simulink model "CoETS_StTrqLimCalc"  (R2016b)
settings: configuration reference "CodeGenConfigSet" (kept outside this file)
values from neighbouring files (symbols this model uses):
  CoETS_nTrqRatMin_C = Calibration.Parameter    [init_CoETS_StTrqLimCalc.m]    (also in init_CoETS_StTrqLimCalc_SIL.m = Simulink.Parameter)
  CoETS_trqDiffMaxLim_C = Calibration.Parameter    [init_CoETS_StTrqLimCalc.m]    (also in init_CoETS_StTrqLimCalc_SIL.m = Simulink.Parameter)
  CoETS_trqInrCurrMinLim_C = Calibration.Parameter    [init_CoETS_StTrqLimCalc.m]    (also in init_CoETS_StTrqLimCalc_SIL.m = Simulink.Parameter)
  PRC_100 = fi(100,Prc_100_rate)    [init_CoETS_StTrqLimCalc.m]    (also in init_CoETS_StTrqLimCalc_SIL.m)
  PRC_ZERO = fi(0,Prc_100_rate)    [init_CoETS_StTrqLimCalc.m]    (also in init_CoETS_StTrqLimCalc_SIL.m)
  Rail_stLimDetSetPoint_C = Calibration.Parameter    [init_CoETS_StTrqLimCalc.m]    (also in init_CoETS_StTrqLimCalc_SIL.m = Simulink.Parameter)
libraries: simulink x68, CXLib x2
settings Model: Creator=Wollf  LastModifiedBy=Wollf
settings ConfigSetRef: SourceLocation=Base Workspace

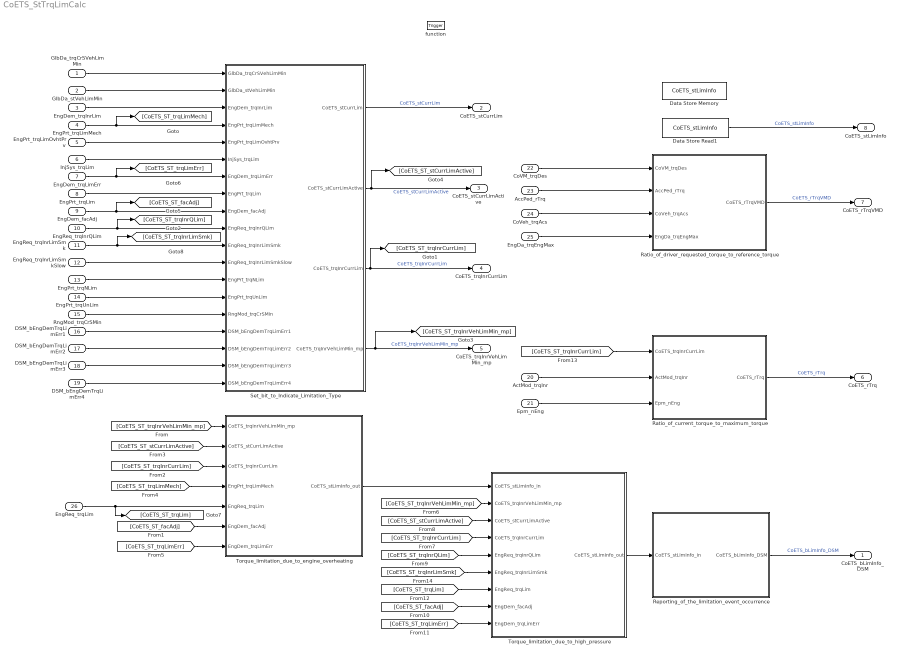
== system CoETS_StTrqLimCalc ==
  GlbDa_trqCrSVehLimMin : Inport  Tag=Nm  Description=current limitation torque from GlbDa on torque level crankshaft  OutMin=-3276.8  OutMax=3276.7  OutDataTypeStr=Trq_Nm
  GlbDa_stVehLimMin : Inport  Description=Current limitation state from GlbDa  Port=2  OutMin=0  OutMax=255  OutDataTypeStr=State_uint8
  EngDem_trqInrLim : Inport  Tag=Nm  Description=Resulting limiting torque (inner engine torque)  Port=3  OutMin=-3276.8  OutMax=3276.7  OutDataTypeStr=Trq_Nm
  EngPrt_trqLimMech : Inport  Tag=Nm  Description=Resulting limiting torque for engine mechanics protection (inner engine torque)  Port=4  OutMin=-3276.8  OutMax=3276.7  OutDataTypeStr=Trq_Nm
  EngPrt_trqLimOvhtPrv : Inport  Tag=Nm  Description=Torque limitation value for engine protection from overheating  Port=5  OutMin=-3276.8  OutMax=3276.7  OutDataTypeStr=Trq_Nm
  InjSys_trqLim : Inport  Tag=Nm  Description=Torque limitation of injection system  Port=6  OutMin=-3276.8  OutMax=3276.7  OutDataTypeStr=Trq_Nm
  EngDem_trqLimErr : Inport  Tag=Nm  Description=Substitute limiting torque in the event of an error  Port=7  OutMin=-3276.8  OutMax=3276.7  OutDataTypeStr=Trq_Nm
  EngPrt_trqLim : Inport  Tag=Nm  Description=Limitation torque for engine mechanic protection by torque limitation (as inner engine torque)  Port=8  OutMin=-3276.8  OutMax=3276.7  OutDataTypeStr=Trq_Nm
  EngDem_facAdj : Inport  Description=EEPROM adjustment value for correction of the limiting torque  Port=9  OutMin=-10  OutMax=10  OutDataTypeStr=Factor
  EngReq_trqInrQLim : Inport  Tag=Nm  Description=Limiting torque due to limitation quantities (except smoke limitation)  Port=10  OutMin=-3276.8  OutMax=3276.7  OutDataTypeStr=Trq_Nm
  EngReq_trqInrLimSmk : Inport  Tag=Nm  Description=Limiting torque smoke limit  Port=11  OutMin=-3276.8  OutMax=3276.7  OutDataTypeStr=Trq_Nm
  EngReq_trqInrLimSmkSlow : Inport  Tag=Nm  Description=Limiting torque smoke limit of slow path  Port=12  OutMin=-3276.8  OutMax=3276.7  OutDataTypeStr=Trq_Nm
  EngPrt_trqNLim : Inport  Tag=Nm  Description=Limiting torque for protection from excessive engine speed  Port=13  OutMin=-3276.8  OutMax=3276.7  OutDataTypeStr=Trq_Nm
  EngPrt_trqUnLim : Inport  Tag=Nm  Description=Enabled torque from the maximum power manager  Port=14  OutMin=-3276.8  OutMax=3276.7  OutDataTypeStr=Trq_Nm
  RngMod_trqCrSMin : Inport  Tag=Nm  Description=minimal crankshaft torque  Port=15  OutMin=-3276.8  OutMax=3276.7  OutDataTypeStr=Trq_Nm
  DSM_bEngDemTrqLimErr1 : Inport  Description=FId for Engine demand Torque Limitation due to System error  Port=16  OutMin=0  OutMax=1  OutDataTypeStr=boolean
  DSM_bEngDemTrqLimErr2 : Inport  Description=FId for Engine demand Torque Limitation due to System error  Port=17  OutMin=0  OutMax=1  OutDataTypeStr=boolean
  DSM_bEngDemTrqLimErr3 : Inport  Description=FId for Engine demand Torque Limitation due to System error  Port=18  OutMin=0  OutMax=1  OutDataTypeStr=boolean
  DSM_bEngDemTrqLimErr4 : Inport  Description=FId for Engine demand Torque Limitation due to System error  Port=19  OutMin=0  OutMax=1  OutDataTypeStr=boolean
  ActMod_trqInr : Inport  Tag=Nm  Description=Current, back-calculated inner engine torque  Port=20  OutMin=-3276.8  OutMax=3276.7  OutDataTypeStr=Trq_Nm
  Epm_nEng : Inport  Tag=rpm  Description=Engine speed  Port=21  OutMin=0  OutMax=6000  OutDataTypeStr=EngSpeed_rpm
  CoVM_trqDes : Inport  Tag=Nm  Description=Propulsion torque order after ESP-torque intervention coordination (wheel torque)  Port=22  OutMin=-3000  OutMax=3000  OutDataTypeStr=Trq_Nm
  AccPed_rTrq : Inport  Description=Total drive train ratio of engine - wheel  Port=23  OutMin=-327  OutMax=327  OutDataTypeStr=TransRatio
  CoVeh_trqAcs : Inport  Tag=Nm  Description=message for demand of accessories  Port=24  OutMin=-3276.8  OutMax=3276.7  OutDataTypeStr=Trq_Nm
  EngDa_trqEngMax : Inport  Tag=Nm  Description=Maximum engine output torque  Port=25  OutMin=-3276.8  OutMax=3276.7  OutDataTypeStr=Trq_Nm
  EngReq_trqLim : Inport  Tag=Nm  Description=Resulting limiting torque from engine specifications  Port=26  OutMin=-3276.8  OutMax=3276.7  OutDataTypeStr=Trq_Nm
  function : TriggerPort  TriggerType=function-call  VariantControl=Variant
  Data Store Memory : DataStoreMemory  DataStoreName=CoETS_stLimInfo  ReadBeforeWriteMsg=warning  WriteAfterWriteMsg=warning  WriteAfterReadMsg=warning  ShowAdditionalParam=off
  Data Store Read1 : DataStoreRead  DataStoreName=CoETS_stLimInfo
  Ratio_of_current_torque_to_maximum_torque : Subsystem
  Ratio_of_driver_requested_torque_to_reference_torque : Subsystem
  Reporting_of_the_limitation_event_occurrence : Subsystem
  Set_bit_to_Indicate_Limitation_Type : Subsystem
  Torque_limitation_due_to_engine_overheating : Subsystem
  Torque_limitation_due_to_high_pressure : Subsystem
  CoETS_bLimInfo_DSM : Outport  Description=DFC of CoETS_bLimInfo  OutMin=0  OutMax=1  OutDataTypeStr=boolean
  CoETS_stCurrLim : Outport  Description=status word for type of lowest limitations  Port=2  OutMin=0  OutMax=65535  OutDataTypeStr=State_uint16
  CoETS_stCurrLimActive : Outport  Description=status of active minimum of limitation torques  Port=3  OutMin=0  OutMax=65535  OutDataTypeStr=State_uint16
  CoETS_trqInrCurrLim : Outport  Tag=Nm  Description=Current lowest limitation torque (inner engine torque)  Port=4  OutMin=-3276.8  OutMax=3276.7  OutDataTypeStr=Trq_Nm
  CoETS_trqInrVehLimMin_mp : Outport  Tag=Nm  Description="Coordinated limitation torque of vehicle functions  (inner torque)"  Port=5  OutMin=-3276.8  OutMax=3276.7  OutDataTypeStr=Trq_Nm
  CoETS_rTrq : Outport  Tag=%  Description=Calculated load value  Port=6  OutMin=-300  OutMax=300  OutDataTypeStr=Prc_100_rate
  CoETS_rTrqVMD : Outport  Tag=%  Description=Ratio of driver requested torque to engine reference torque  Port=7  OutMin=-300  OutMax=300  OutDataTypeStr=Prc_100_rate
  CoETS_stLimInfo : Outport  Description=Status information on working torque limitation  Port=8  OutMin=0  OutMax=255  OutDataTypeStr=State_uint8
  wires:
  RngMod_trqCrSMin/1 -> Set_bit_to_Indicate_Limitation_Type/15(RngMod_trqCrSMin)
  AccPed_rTrq/1 -> Ratio_of_driver_requested_torque_to_reference_torque/2(AccPed_rTrq)
  Ratio_of_driver_requested_torque_to_reference_torque/1("CoETS_rTrqVMD ") -> CoETS_rTrqVMD/1  "CoETS_rTrqVMD"
  CoVM_trqDes/1 -> Ratio_of_driver_requested_torque_to_reference_torque/1(CoVM_trqDes)
  EngDa_trqEngMax/1 -> Ratio_of_driver_requested_torque_to_reference_torque/4(EngDa_trqEngMax)
  CoVeh_trqAcs/1 -> Ratio_of_driver_requested_torque_to_reference_torque/3(CoVeh_trqAcs)
  Ratio_of_current_torque_to_maximum_torque/1(CoETS_rTrq) -> CoETS_rTrq/1  "CoETS_rTrq"
  EngReq_trqInrLimSmk/1 -> Set_bit_to_Indicate_Limitation_Type/11(EngReq_trqInrLimSmk), [CoETS_ST_trqInrLimSmk]
  EngPrt_trqLim/1 -> Set_bit_to_Indicate_Limitation_Type/8(EngPrt_trqLim)
  InjSys_trqLim/1 -> Set_bit_to_Indicate_Limitation_Type/6("InjSys_trqLim ")
  EngDem_facAdj/1 -> Set_bit_to_Indicate_Limitation_Type/9(EngDem_facAdj), [CoETS_ST_facAdj]
  EngDem_trqLimErr/1 -> Set_bit_to_Indicate_Limitation_Type/7(EngDem_trqLimErr), [CoETS_ST_trqLimErr]
  EngPrt_trqUnLim/1 -> Set_bit_to_Indicate_Limitation_Type/14(EngPrt_trqUnLim)
  EngPrt_trqNLim/1 -> Set_bit_to_Indicate_Limitation_Type/13(EngPrt_trqNLim)
  Set_bit_to_Indicate_Limitation_Type/2(CoETS_stCurrLimActive) -> CoETS_stCurrLimActive/1, [CoETS_ST_stCurrLimActive]  "CoETS_stCurrLimActive"
  EngReq_trqInrLimSmkSlow/1 -> Set_bit_to_Indicate_Limitation_Type/12(EngReq_trqInrLimSmkSlow)
  GlbDa_stVehLimMin/1 -> Set_bit_to_Indicate_Limitation_Type/2(GlbDa_stVehLimMin)
  EngReq_trqInrQLim/1 -> Set_bit_to_Indicate_Limitation_Type/10(EngReq_trqInrQLim), [CoETS_ST_trqInrQLim]
  EngDem_trqInrLim/1 -> Set_bit_to_Indicate_Limitation_Type/3(EngDem_trqInrLim)
  GlbDa_trqCrSVehLimMin/1 -> Set_bit_to_Indicate_Limitation_Type/1(GlbDa_trqCrSVehLimMin)
  EngPrt_trqLimOvhtPrv/1 -> Set_bit_to_Indicate_Limitation_Type/5("EngPrt_trqLimOvhtPrv ")
  Set_bit_to_Indicate_Limitation_Type/1(CoETS_stCurrLim) -> CoETS_stCurrLim/1  "CoETS_stCurrLim"
  EngPrt_trqLimMech/1 -> Set_bit_to_Indicate_Limitation_Type/4(EngPrt_trqLimMech), [CoETS_ST_trqLimMech]
  [CoETS_ST_trqInrCurrLim] -> Ratio_of_current_torque_to_maximum_torque/1(CoETS_trqInrCurrLim)
  Set_bit_to_Indicate_Limitation_Type/3(CoETS_trqInrCurrLim) -> CoETS_trqInrCurrLim/1, [CoETS_ST_trqInrCurrLim]  "CoETS_trqInrCurrLim"
  [CoETS_ST_trqInrCurrLim] -> Torque_limitation_due_to_engine_overheating/3(CoETS_trqInrCurrLim)
  Set_bit_to_Indicate_Limitation_Type/4(CoETS_trqInrVehLimMin_mp) -> CoETS_trqInrVehLimMin_mp/1, [CoETS_ST_trqInrVehLimMin_mp]  "CoETS_trqInrVehLimMin_mp"
  [CoETS_ST_trqInrVehLimMin_mp] -> Torque_limitation_due_to_engine_overheating/1(CoETS_trqInrVehLimMin_mp)
  [CoETS_ST_stCurrLimActive] -> Torque_limitation_due_to_engine_overheating/2(CoETS_stCurrLimActive)
  [CoETS_ST_trqLimMech] -> Torque_limitation_due_to_engine_overheating/4(EngPrt_trqLimMech)
  EngReq_trqLim/1 -> Torque_limitation_due_to_engine_overheating/5(EngReq_trqLim), [CoETS_ST_trqLim]
  [CoETS_ST_facAdj] -> Torque_limitation_due_to_engine_overheating/6(EngDem_facAdj)
  [CoETS_ST_trqLimErr] -> Torque_limitation_due_to_engine_overheating/7(EngDem_trqLimErr)
  [CoETS_ST_trqInrVehLimMin_mp] -> Torque_limitation_due_to_high_pressure/2(CoETS_trqInrVehLimMin_mp)
  [CoETS_ST_stCurrLimActive] -> Torque_limitation_due_to_high_pressure/3(CoETS_stCurrLimActive)
  [CoETS_ST_trqInrCurrLim] -> Torque_limitation_due_to_high_pressure/4(CoETS_trqInrCurrLim)
  [CoETS_ST_trqInrQLim] -> Torque_limitation_due_to_high_pressure/5(EngReq_trqInrQLim)
  [CoETS_ST_facAdj] -> Torque_limitation_due_to_high_pressure/8(EngDem_facAdj)
  [CoETS_ST_trqLimErr] -> Torque_limitation_due_to_high_pressure/9(EngDem_trqLimErr)
  [CoETS_ST_trqLim] -> Torque_limitation_due_to_high_pressure/7(EngReq_trqLim)
  [CoETS_ST_trqInrLimSmk] -> Torque_limitation_due_to_high_pressure/6(EngReq_trqInrLimSmk)
  Torque_limitation_due_to_engine_overheating/1("CoETS_stLimInfo_out ") -> Torque_limitation_due_to_high_pressure/1(CoETS_stLimInfo_in)
  Torque_limitation_due_to_high_pressure/1("CoETS_stLimInfo_out ") -> Reporting_of_the_limitation_event_occurrence/1(CoETS_stLimInfo_in)
  Reporting_of_the_limitation_event_occurrence/1(CoETS_bLimInfo_DSM) -> CoETS_bLimInfo_DSM/1  "CoETS_bLimInfo_DSM"
  DSM_bEngDemTrqLimErr1/1 -> Set_bit_to_Indicate_Limitation_Type/16(DSM_bEngDemTrqLimErr1)
  DSM_bEngDemTrqLimErr2/1 -> Set_bit_to_Indicate_Limitation_Type/17(DSM_bEngDemTrqLimErr2)
  DSM_bEngDemTrqLimErr3/1 -> Set_bit_to_Indicate_Limitation_Type/18(DSM_bEngDemTrqLimErr3)
  DSM_bEngDemTrqLimErr4/1 -> Set_bit_to_Indicate_Limitation_Type/19(DSM_bEngDemTrqLimErr4)
  ActMod_trqInr/1 -> Ratio_of_current_torque_to_maximum_torque/2(ActMod_trqInr)
  Epm_nEng/1 -> Ratio_of_current_torque_to_maximum_torque/3(Epm_nEng)
  Data Store Read1/1 -> CoETS_stLimInfo/1  "CoETS_stLimInfo"

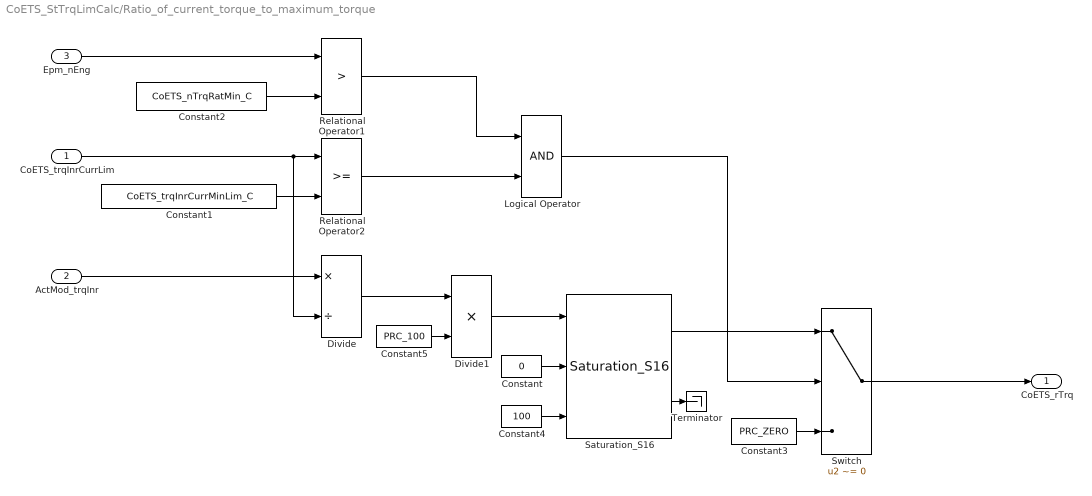
== system CoETS_StTrqLimCalc/Ratio_of_current_torque_to_maximum_torque ==
  CoETS_trqInrCurrLim : Inport
  ActMod_trqInr : Inport  Port=2
  Epm_nEng : Inport  Port=3
  Constant : Constant  Value=0  OutDataTypeStr=Inherit: Inherit via back propagation
  Constant1 : Constant  Value=CoETS_trqInrCurrMinLim_C
  Constant2 : Constant  Value=CoETS_nTrqRatMin_C
  Constant3 : Constant  Value=PRC_ZERO  OutDataTypeStr=Inherit: Inherit via back propagation
  Constant4 : Constant  Value=100  OutDataTypeStr=Inherit: Inherit via back propagation
  Constant5 : Constant  Value=PRC_100  OutDataTypeStr=uint8
  Divide : Product  Inputs=*/  OutDataTypeStr=Accpedal_rate  SaturateOnIntegerOverflow=on
  Divide1 : Product  Inputs=**  OutDataTypeStr=Inherit: Inherit via back propagation  SaturateOnIntegerOverflow=on
  Logical Operator : Logic  OutDataTypeStr=boolean
  Relational Operator1 : RelationalOperator  Operator=>  OutDataTypeStr=boolean  RndMeth=Nearest  InputSameDT=on
  Relational Operator2 : RelationalOperator  OutDataTypeStr=boolean  RndMeth=Nearest  InputSameDT=on
  Saturation_S16 : CXLib/Saturation_S16
  Switch : Switch  Criteria=u2 ~= 0  SaturateOnIntegerOverflow=on  InputSameDT=on
  Terminator : Terminator
  CoETS_rTrq : Outport
  wires:
  CoETS_trqInrCurrLim/1 -> Relational Operator2/1, Divide/2
  Constant2/1 -> Relational Operator1/2
  Epm_nEng/1 -> Relational Operator1/1
  Constant1/1 -> Relational Operator2/2
  Relational Operator1/1 -> Logical Operator/1
  Relational Operator2/1 -> Logical Operator/2
  Logical Operator/1 -> Switch/2
  Constant3/1 -> Switch/3
  ActMod_trqInr/1 -> Divide/1
  Divide/1 -> Divide1/1
  Constant/1 -> Saturation_S16/2
  Constant4/1 -> Saturation_S16/3
  Saturation_S16/2 -> Terminator/1
  Saturation_S16/1 -> Switch/1
  Switch/1 -> CoETS_rTrq/1
  Constant5/1 -> Divide1/2
  Divide1/1 -> Saturation_S16/1

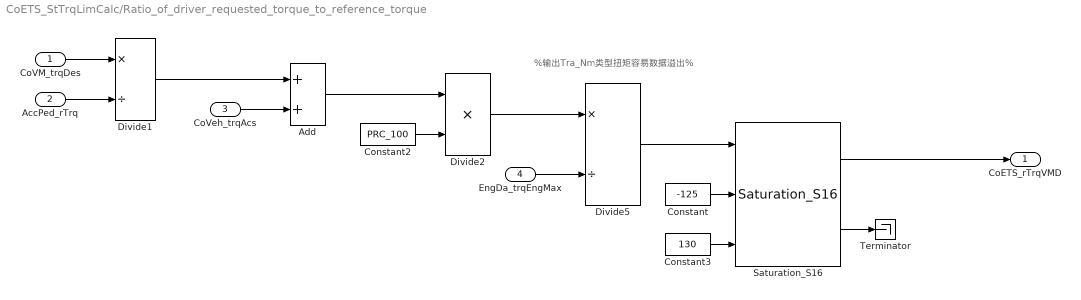
== system CoETS_StTrqLimCalc/Ratio_of_driver_requested_torque_to_reference_torque ==
  note: %输出Tra_Nm类型扭矩容易数据溢出%
  CoVM_trqDes : Inport
  AccPed_rTrq : Inport  Port=2
  CoVeh_trqAcs : Inport  Port=3
  EngDa_trqEngMax : Inport  Port=4
  Add : Sum  SaturateOnIntegerOverflow=on  InputSameDT=on
  Constant : Constant  Value=-125  OutDataTypeStr=Inherit: Inherit via back propagation
  Constant2 : Constant  Value=PRC_100  OutDataTypeStr=uint8
  Constant3 : Constant  Value=130  OutDataTypeStr=Inherit: Inherit via back propagation
  Divide1 : Product  Inputs=*/  OutDataTypeStr=Trq_Nm  SaturateOnIntegerOverflow=on
  Divide2 : Product  Inputs=**  OutDataTypeStr=int32  SaturateOnIntegerOverflow=on
  Divide5 : Product  Inputs=*/  OutDataTypeStr=Inherit: Inherit via back propagation  SaturateOnIntegerOverflow=on
  Saturation_S16 : CXLib/Saturation_S16
  Terminator : Terminator
  "CoETS_rTrqVMD " : Outport
  wires:
  AccPed_rTrq/1 -> Divide1/2
  Divide1/1 -> Add/1
  CoVeh_trqAcs/1 -> Add/2
  Add/1 -> Divide2/1
  Constant2/1 -> Divide2/2
  EngDa_trqEngMax/1 -> Divide5/2
  Divide5/1 -> Saturation_S16/1
  Constant/1 -> Saturation_S16/2
  Constant3/1 -> Saturation_S16/3
  Saturation_S16/1 -> "CoETS_rTrqVMD "/1
  Saturation_S16/2 -> Terminator/1
  CoVM_trqDes/1 -> Divide1/1
  Divide2/1 -> Divide5/1

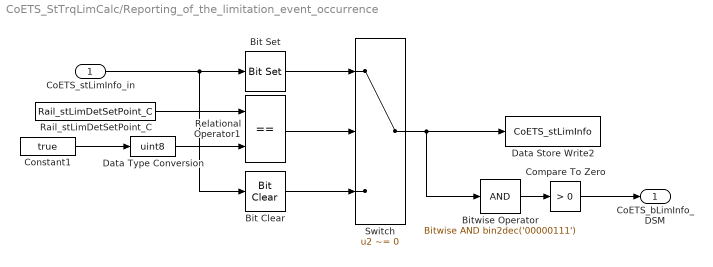
== system CoETS_StTrqLimCalc/Reporting_of_the_limitation_event_occurrence ==
  CoETS_stLimInfo_in : Inport
  Bit Clear : simulink/Logic and Bit Operations/Bit Clear  iBit=2
  Bit Set : simulink/Logic and Bit Operations/Bit Set  iBit=2
  Bitwise Operator : simulink/Logic and Bit Operations/Bitwise Operator  logicop=AND  UseBitMask=on  BitMask=bin2dec('00000111')  BitMaskRealWorld=Stored Integer
  Compare To Zero : simulink/Logic and Bit Operations/Compare To Zero  relop=>  OutDataTypeStr=boolean
  Constant1 : Constant  Value=true  OutDataTypeStr=boolean
  Data Store Write2 : DataStoreWrite  DataStoreName=CoETS_stLimInfo
  Data Type Conversion : DataTypeConversion  OutDataTypeStr=uint8
  Rail_stLimDetSetPoint_C : Constant  Value=Rail_stLimDetSetPoint_C
  Relational Operator1 : RelationalOperator  Operator===  OutDataTypeStr=boolean  RndMeth=Nearest  InputSameDT=on
  Switch : Switch  Criteria=u2 ~= 0  InputSameDT=on
  CoETS_bLimInfo_DSM : Outport
  wires:
  Constant1/1 -> Data Type Conversion/1
  Relational Operator1/1 -> Switch/2
  CoETS_stLimInfo_in/1 -> Bit Clear/1, Bit Set/1
  Bit Set/1 -> Switch/1
  Bit Clear/1 -> Switch/3
  Rail_stLimDetSetPoint_C/1 -> Relational Operator1/1
  Switch/1 -> Data Store Write2/1, Bitwise Operator/1
  Bitwise Operator/1 -> Compare To Zero/1
  Compare To Zero/1 -> CoETS_bLimInfo_DSM/1
  Data Type Conversion/1 -> Relational Operator1/2

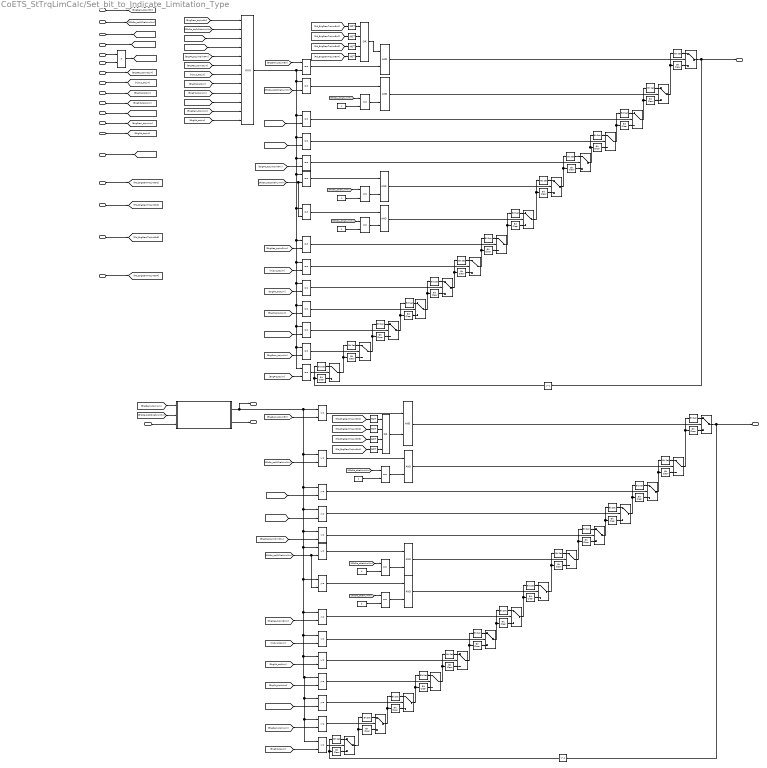
== system CoETS_StTrqLimCalc/Set_bit_to_Indicate_Limitation_Type ==
  note: FId must be a uint16 constant
  GlbDa_trqCrSVehLimMin : Inport
  GlbDa_stVehLimMin : Inport  Port=2
  EngDem_trqInrLim : Inport  Port=3
  EngPrt_trqLimMech : Inport  Port=4
  "EngPrt_trqLimOvhtPrv " : Inport  Port=5
  "InjSys_trqLim " : Inport  Port=6
  EngDem_trqLimErr : Inport  Port=7
  EngPrt_trqLim : Inport  Port=8
  EngDem_facAdj : Inport  Port=9
  EngReq_trqInrQLim : Inport  Port=10
  EngReq_trqInrLimSmk : Inport  Port=11
  EngReq_trqInrLimSmkSlow : Inport  Port=12
  EngPrt_trqNLim : Inport  Port=13
  EngPrt_trqUnLim : Inport  Port=14
  RngMod_trqCrSMin : Inport  Port=15
  DSM_bEngDemTrqLimErr1 : Inport  Port=16
  DSM_bEngDemTrqLimErr2 : Inport  Port=17
  DSM_bEngDemTrqLimErr3 : Inport  Port=18
  DSM_bEngDemTrqLimErr4 : Inport  Port=19
  Bit Clear1 : simulink/Logic and Bit Operations/Bit Clear  iBit=0
  Bit Clear12 : simulink/Logic and Bit Operations/Bit Clear  iBit=10
  Bit Clear14 : simulink/Logic and Bit Operations/Bit Clear  iBit=11
  Bit Clear16 : simulink/Logic and Bit Operations/Bit Clear  iBit=12
  Bit Clear18 : simulink/Logic and Bit Operations/Bit Clear  iBit=13
  Bit Clear2 : simulink/Logic and Bit Operations/Bit Clear  iBit=6
  Bit Clear20 : simulink/Logic and Bit Operations/Bit Clear  iBit=14
  Bit Clear3 : simulink/Logic and Bit Operations/Bit Clear  iBit=1
  Bit Clear4 : simulink/Logic and Bit Operations/Bit Clear  iBit=2
  Bit Clear41 : simulink/Logic and Bit Operations/Bit Clear  iBit=0
  Bit Clear44 : simulink/Logic and Bit Operations/Bit Clear  iBit=10
  Bit Clear46 : simulink/Logic and Bit Operations/Bit Clear  iBit=11
  Bit Clear48 : simulink/Logic and Bit Operations/Bit Clear  iBit=12
  Bit Clear5 : simulink/Logic and Bit Operations/Bit Clear  iBit=3
  Bit Clear50 : simulink/Logic and Bit Operations/Bit Clear  iBit=13
  Bit Clear52 : simulink/Logic and Bit Operations/Bit Clear  iBit=6
  Bit Clear53 : simulink/Logic and Bit Operations/Bit Clear  iBit=14
  Bit Clear54 : simulink/Logic and Bit Operations/Bit Clear  iBit=1
  Bit Clear55 : simulink/Logic and Bit Operations/Bit Clear  iBit=2
  Bit Clear56 : simulink/Logic and Bit Operations/Bit Clear  iBit=3
  Bit Clear57 : simulink/Logic and Bit Operations/Bit Clear  iBit=5
  Bit Clear58 : simulink/Logic and Bit Operations/Bit Clear  iBit=7
  Bit Clear59 : simulink/Logic and Bit Operations/Bit Clear  iBit=8
  Bit Clear6 : simulink/Logic and Bit Operations/Bit Clear  iBit=5
  Bit Clear60 : simulink/Logic and Bit Operations/Bit Clear  iBit=9
  Bit Clear7 : simulink/Logic and Bit Operations/Bit Clear  iBit=7
  Bit Clear8 : simulink/Logic and Bit Operations/Bit Clear  iBit=8
  Bit Clear9 : simulink/Logic and Bit Operations/Bit Clear  iBit=9
  Bit Set1 : simulink/Logic and Bit Operations/Bit Set  iBit=0
  Bit Set10 : simulink/Logic and Bit Operations/Bit Set  iBit=10
  Bit Set11 : simulink/Logic and Bit Operations/Bit Set  iBit=11
  Bit Set12 : simulink/Logic and Bit Operations/Bit Set  iBit=12
  Bit Set13 : simulink/Logic and Bit Operations/Bit Set  iBit=13
  Bit Set14 : simulink/Logic and Bit Operations/Bit Set  iBit=14
  Bit Set15 : simulink/Logic and Bit Operations/Bit Set  iBit=9
  Bit Set16 : simulink/Logic and Bit Operations/Bit Set  iBit=10
  Bit Set17 : simulink/Logic and Bit Operations/Bit Set  iBit=6
  Bit Set18 : simulink/Logic and Bit Operations/Bit Set  iBit=1
  Bit Set19 : simulink/Logic and Bit Operations/Bit Set  iBit=2
  Bit Set2 : simulink/Logic and Bit Operations/Bit Set  iBit=6
  Bit Set20 : simulink/Logic and Bit Operations/Bit Set  iBit=3
  Bit Set21 : simulink/Logic and Bit Operations/Bit Set  iBit=5
  Bit Set22 : simulink/Logic and Bit Operations/Bit Set  iBit=7
  Bit Set23 : simulink/Logic and Bit Operations/Bit Set  iBit=8
  Bit Set24 : simulink/Logic and Bit Operations/Bit Set  iBit=0
  Bit Set25 : simulink/Logic and Bit Operations/Bit Set  iBit=11
  Bit Set26 : simulink/Logic and Bit Operations/Bit Set  iBit=12
  Bit Set27 : simulink/Logic and Bit Operations/Bit Set  iBit=13
  Bit Set28 : simulink/Logic and Bit Operations/Bit Set  iBit=14
  Bit Set3 : simulink/Logic and Bit Operations/Bit Set  iBit=1
  Bit Set4 : simulink/Logic and Bit Operations/Bit Set  iBit=2
  Bit Set5 : simulink/Logic and Bit Operations/Bit Set  iBit=3
  Bit Set6 : simulink/Logic and Bit Operations/Bit Set  iBit=5
  Bit Set7 : simulink/Logic and Bit Operations/Bit Set  iBit=7
  Bit Set8 : simulink/Logic and Bit Operations/Bit Set  iBit=8
  Bit Set9 : simulink/Logic and Bit Operations/Bit Set  iBit=9
  Constant1 : Constant  OutDataTypeStr=uint8
  Constant12 : Constant  OutDataTypeStr=uint8
  Constant13 : Constant  Value=4  OutDataTypeStr=uint8
  Constant14 : Constant  Value=2  OutDataTypeStr=Inherit: Inherit via back propagation
  Constant2 : Constant  Value=4  OutDataTypeStr=uint8
  Constant3 : Constant  Value=2  OutDataTypeStr=uint8
  Delay : Delay  DelayLength=1  InitialCondition=0
  Delay2 : Delay  DelayLength=1  InitialCondition=0
  Determining_the_current_minimum_of_all_torque_limitations : Subsystem
  Divide : Product  Inputs=**  OutDataTypeStr=Inherit: Inherit via back propagation  SaturateOnIntegerOverflow=on
  Logical Operator{,1..2,4,6..8,16} (8 alike) : Logic  OutDataTypeStr=boolean
  Logical Operator{5,9..11,13..14,17,19} (8 alike) : Logic  Operator=NOT  OutDataTypeStr=boolean
  Logical Operator12 : Logic  Operator=OR  Inputs=4  OutDataTypeStr=boolean
  Logical Operator15 : Logic  Operator=OR  Inputs=4  OutDataTypeStr=boolean
  MinMax : MinMax  Inputs=12  SaturateOnIntegerOverflow=on  InputSameDT=on
  Relational Operator{1..5,7,9,11..17} (14 alike) : RelationalOperator  OutDataTypeStr=boolean  RndMeth=Nearest  InputSameDT=on
  Relational Operator{6,8,10,18..34} (20 alike) : RelationalOperator  Operator===  OutDataTypeStr=boolean  RndMeth=Nearest  InputSameDT=on
  Switch{1..14,29..42} (28 alike) : Switch  Criteria=u2 ~= 0  InputSameDT=on
  CoETS_stCurrLim : Outport
  CoETS_stCurrLimActive : Outport  Port=2
  CoETS_trqInrCurrLim : Outport  Port=3
  CoETS_trqInrVehLimMin_mp : Outport  Port=4
  wires:
  EngDem_trqLimErr/1 -> [EngDem_trqLimErr]
  Bit Set1/1 -> Switch1/1
  Bit Clear1/1 -> Switch1/3
  Logical Operator16/1 -> Switch1/2
  Switch1/1 -> Delay/1, CoETS_stCurrLim/1
  Logical Operator/1 -> Switch3/2
  Bit Set3/1 -> Switch3/1
  Bit Clear3/1 -> Switch3/3
  Bit Set4/1 -> Switch4/1
  Bit Clear4/1 -> Switch4/3
  Relational Operator4/1 -> Switch4/2
  Relational Operator1/1 -> Switch5/2
  Bit Set5/1 -> Switch5/1
  Bit Clear5/1 -> Switch5/3
  Bit Set6/1 -> Switch6/1
  Bit Clear6/1 -> Switch6/3
  Relational Operator5/1 -> Switch6/2
  GlbDa_trqCrSVehLimMin/1 -> [GlbDa_trqCrSVehLimMin]
  Relational Operator3/1 -> Logical Operator/1
  Relational Operator6/1 -> Logical Operator/2
  GlbDa_stVehLimMin/1 -> [GlbDa_stVehLimMin]
  Constant1/1 -> Relational Operator6/2
  EngPrt_trqLimMech/1 -> [EngPrt_trqLimMech]
  EngReq_trqInrLimSmk/1 -> [EngReq_trqInrLimSmk]
  Bit Clear2/1 -> Switch2/3
  Logical Operator1/1 -> Switch2/2
  Relational Operator8/1 -> Logical Operator1/2
  Relational Operator7/1 -> Logical Operator1/1
  Constant2/1 -> Relational Operator8/2
  Bit Set2/1 -> Switch2/1
  Bit Clear7/1 -> Switch7/3
  Logical Operator2/1 -> Switch7/2
  Relational Operator10/1 -> Logical Operator2/2
  Relational Operator9/1 -> Logical Operator2/1
  Bit Set7/1 -> Switch7/1
  Constant3/1 -> Relational Operator10/2
  Bit Set8/1 -> Switch8/1
  Bit Clear8/1 -> Switch8/3
  Relational Operator11/1 -> Switch8/2
  Bit Clear9/1 -> Switch9/3
  Relational Operator12/1 -> Switch9/2
  "InjSys_trqLim "/1 -> [InjSys_trqLim]
  Bit Set15/1 -> Switch9/1
  Bit Clear12/1 -> Switch10/3
  Relational Operator13/1 -> Switch10/2
  EngPrt_trqNLim/1 -> [EngPrt_trqNLim]
  Bit Set16/1 -> Switch10/1
  Bit Clear14/1 -> Switch11/3
  Relational Operator14/1 -> Switch11/2
  EngPrt_trqUnLim/1 -> [EngPrt_trqUnLim]
  Bit Set25/1 -> Switch11/1
  Determining_the_current_minimum_of_all_torque_limitations/1(CoETS_trqInrCurrLim) -> Relational Operator7/1, Relational Operator17/1, Relational Operator16/1, Relational Operator15/1, Relational Operator14/1, Relational Operator13/1, Relational Operator12/1, Relational Operator11/1, Relational Operator9/1, Relational Operator5/1, Relational Operator1/1, Relational Operator4/1, Relational Operator3/1, Relational Operator2/1, CoETS_trqInrCurrLim/1
  Bit Clear16/1 -> Switch12/3
  Relational Operator15/1 -> Switch12/2
  EngReq_trqInrLimSmkSlow/1 -> [EngReq_trqInrLimSmkSlow]
  Bit Set26/1 -> Switch12/1
  Bit Clear18/1 -> Switch13/3
  Relational Operator16/1 -> Switch13/2
  Bit Set27/1 -> Switch13/1
  Bit Clear20/1 -> Switch14/3
  Relational Operator17/1 -> Switch14/2
  Bit Set28/1 -> Switch14/1
  EngDem_trqInrLim/1 -> [EngDem_trqInrLim]
  EngPrt_trqLim/1 -> [EngPrt_trqLim]
  EngDem_facAdj/1 -> Divide/2
  "EngPrt_trqLimOvhtPrv "/1 -> Divide/1
  Divide/1 -> [EngPrt_trqLimOvhtPrv]
  Switch14/1 -> Bit Set27/1, Bit Clear18/1
  Switch13/1 -> Bit Set26/1, Bit Clear16/1
  Switch12/1 -> Bit Set25/1, Bit Clear14/1
  Switch11/1 -> Bit Set16/1, Bit Clear12/1
  Switch10/1 -> Bit Set15/1, Bit Clear9/1
  Switch9/1 -> Bit Clear8/1, Bit Set8/1
  Switch8/1 -> Bit Set7/1, Bit Clear7/1
  Switch7/1 -> Bit Clear2/1, Bit Set2/1
  Switch2/1 -> Bit Clear6/1, Bit Set6/1
  Switch6/1 -> Bit Clear5/1, Bit Set5/1
  Switch5/1 -> Bit Clear4/1, Bit Set4/1
  Switch4/1 -> Bit Clear3/1, Bit Set3/1
  Switch3/1 -> Bit Clear1/1, Bit Set1/1
  Delay/1 -> Bit Set28/1, Bit Clear20/1
  Bit Set24/1 -> Switch29/1
  Bit Clear41/1 -> Switch29/3
  Logical Operator4/1 -> Switch29/2
  Switch29/1 -> CoETS_stCurrLimActive/1, Delay2/1
  Logical Operator6/1 -> Switch36/2
  Bit Set18/1 -> Switch36/1
  Bit Clear54/1 -> Switch36/3
  Bit Set19/1 -> Switch37/1
  Bit Clear55/1 -> Switch37/3
  Relational Operator21/1 -> Switch37/2
  Relational Operator22/1 -> Switch38/2
  Bit Set20/1 -> Switch38/1
  Bit Clear56/1 -> Switch38/3
  Bit Set21/1 -> Switch39/1
  Bit Clear57/1 -> Switch39/3
  Relational Operator23/1 -> Switch39/2
  Relational Operator19/1 -> Logical Operator6/1
  Relational Operator20/1 -> Logical Operator6/2
  Bit Clear52/1 -> Switch35/3
  Logical Operator7/1 -> Switch35/2
  Relational Operator25/1 -> Logical Operator7/2
  Relational Operator24/1 -> Logical Operator7/1
  Bit Set17/1 -> Switch35/1
  Bit Clear58/1 -> Switch40/3
  Logical Operator8/1 -> Switch40/2
  Relational Operator27/1 -> Logical Operator8/2
  Relational Operator26/1 -> Logical Operator8/1
  Bit Set22/1 -> Switch40/1
  Bit Set23/1 -> Switch41/1
  Bit Clear59/1 -> Switch41/3
  Relational Operator28/1 -> Switch41/2
  Bit Clear60/1 -> Switch42/3
  Relational Operator29/1 -> Switch42/2
  Bit Set9/1 -> Switch42/1
  Bit Clear44/1 -> Switch30/3
  Relational Operator30/1 -> Switch30/2
  Bit Set10/1 -> Switch30/1
  Bit Clear46/1 -> Switch31/3
  Relational Operator31/1 -> Switch31/2
  Bit Set11/1 -> Switch31/1
  Bit Clear48/1 -> Switch32/3
  Relational Operator32/1 -> Switch32/2
  Bit Set12/1 -> Switch32/1
  Bit Clear50/1 -> Switch33/3
  Relational Operator33/1 -> Switch33/2
  Bit Set13/1 -> Switch33/1
  Bit Clear53/1 -> Switch34/3
  Relational Operator34/1 -> Switch34/2
  Bit Set14/1 -> Switch34/1
  Switch34/1 -> Bit Set13/1, Bit Clear50/1
  Switch33/1 -> Bit Set12/1, Bit Clear48/1
  Switch32/1 -> Bit Set11/1, Bit Clear46/1
  Switch31/1 -> Bit Set10/1, Bit Clear44/1
  Switch30/1 -> Bit Set9/1, Bit Clear60/1
  Switch42/1 -> Bit Clear59/1, Bit Set23/1
  Switch41/1 -> Bit Set22/1, Bit Clear58/1
  Switch40/1 -> Bit Clear52/1, Bit Set17/1
  Switch35/1 -> Bit Set21/1, Bit Clear57/1
  Switch39/1 -> Bit Clear56/1, Bit Set20/1
  Switch38/1 -> Bit Clear55/1, Bit Set19/1
  Switch37/1 -> Bit Clear54/1, Bit Set18/1
  Switch36/1 -> Bit Clear41/1, Bit Set24/1
  Delay2/1 -> Bit Set14/1, Bit Clear53/1
  EngReq_trqInrQLim/1 -> [EngReq_trqInrQLim]
  [EngDem_trqLimErr] -> MinMax/1
  [GlbDa_trqCrSVehLimMin] -> MinMax/2
  [GlbDa_stVehLimMin] -> Relational Operator20/1
  [EngReq_trqInrLimSmk] -> MinMax/4
  [EngPrt_trqLimOvhtPrv] -> MinMax/5
  [EngReq_trqInrQLim] -> MinMax/6
  [InjSys_trqLim] -> MinMax/7
  [EngPrt_trqNLim] -> MinMax/8
  [EngPrt_trqUnLim] -> MinMax/9
  [EngReq_trqInrLimSmkSlow] -> MinMax/10
  [EngDem_trqInrLim] -> MinMax/11
  [EngPrt_trqLim] -> MinMax/12
  Relational Operator18/1 -> Logical Operator4/2
  MinMax/1 -> Relational Operator21/1, Relational Operator26/1, Relational Operator34/1, Relational Operator33/1, Relational Operator32/1, Relational Operator31/1, Relational Operator30/1, Relational Operator29/1, Relational Operator28/1, Relational Operator24/1, Relational Operator23/1, Relational Operator22/1, Relational Operator19/1, Relational Operator18/2
  [EngDem_trqLimErr] -> Relational Operator18/1
  [GlbDa_trqCrSVehLimMin] -> Relational Operator19/2
  Constant12/1 -> Relational Operator20/2
  [EngPrt_trqLimMech] -> MinMax/3
  [EngPrt_trqLimMech] -> Relational Operator21/2
  [EngReq_trqInrLimSmk] -> Relational Operator22/2
  [EngPrt_trqLimOvhtPrv] -> Relational Operator23/2
  [GlbDa_trqCrSVehLimMin] -> Relational Operator24/2, Relational Operator26/2
  Constant13/1 -> Relational Operator25/2
  Constant14/1 -> Relational Operator27/2
  [EngReq_trqInrQLim] -> Relational Operator28/2
  [InjSys_trqLim] -> Relational Operator29/2
  [EngPrt_trqNLim] -> Relational Operator30/2
  [EngPrt_trqUnLim] -> Relational Operator31/2
  [EngReq_trqInrLimSmkSlow] -> Relational Operator32/2
  [EngDem_trqInrLim] -> Relational Operator33/2
  [EngPrt_trqLim] -> Relational Operator34/2
  [FId_EngDemTrqLimErr1] -> Logical Operator5/1
  [FId_EngDemTrqLimErr4] -> Logical Operator11/1
  [FId_EngDemTrqLimErr2] -> Logical Operator9/1
  [FId_EngDemTrqLimErr3] -> Logical Operator10/1
  Logical Operator5/1 -> Logical Operator12/1
  Logical Operator9/1 -> Logical Operator12/2
  Logical Operator10/1 -> Logical Operator12/3
  Logical Operator11/1 -> Logical Operator12/4
  Logical Operator12/1 -> Logical Operator4/1
  Relational Operator2/1 -> Logical Operator16/1
  [FId_EngDemTrqLimErr1] -> Logical Operator17/1
  [FId_EngDemTrqLimErr4] -> Logical Operator14/1
  [FId_EngDemTrqLimErr2] -> Logical Operator19/1
  [FId_EngDemTrqLimErr3] -> Logical Operator13/1
  Logical Operator17/1 -> Logical Operator15/1
  Logical Operator19/1 -> Logical Operator15/2
  Logical Operator13/1 -> Logical Operator15/3
  Logical Operator14/1 -> Logical Operator15/4
  Logical Operator15/1 -> Logical Operator16/2
  [GlbDa_stVehLimMin] -> Relational Operator25/1
  [GlbDa_stVehLimMin] -> Relational Operator27/1
  [GlbDa_stVehLimMin] -> Relational Operator6/1
  [GlbDa_stVehLimMin] -> Relational Operator8/1
  [GlbDa_stVehLimMin] -> Relational Operator10/1
  [EngDem_trqLimErr] -> Relational Operator2/2
  [GlbDa_trqCrSVehLimMin] -> Relational Operator3/2
  [GlbDa_trqCrSVehLimMin] -> Relational Operator9/2, Relational Operator7/2
  [EngPrt_trqLimMech] -> Relational Operator4/2
  [EngReq_trqInrLimSmk] -> Relational Operator1/2
  [EngPrt_trqLimOvhtPrv] -> Relational Operator5/2
  [EngReq_trqInrQLim] -> Relational Operator11/2
  [InjSys_trqLim] -> Relational Operator12/2
  [EngPrt_trqNLim] -> Relational Operator13/2
  [EngPrt_trqUnLim] -> Relational Operator14/2
  [EngReq_trqInrLimSmkSlow] -> Relational Operator15/2
  [EngDem_trqInrLim] -> Relational Operator16/2
  [EngPrt_trqLim] -> Relational Operator17/2
  Determining_the_current_minimum_of_all_torque_limitations/2(CoETS_trqInrVehLimMin_mp) -> CoETS_trqInrVehLimMin_mp/1
  RngMod_trqCrSMin/1 -> Determining_the_current_minimum_of_all_torque_limitations/3(RngMod_trqCrSMin)
  [EngDem_trqInrLim] -> Determining_the_current_minimum_of_all_torque_limitations/1(EngDem_trqInrLim)
  [GlbDa_trqCrSVehLimMin] -> Determining_the_current_minimum_of_all_torque_limitations/2(GlbDa_trqCrSVehLimMin)
  DSM_bEngDemTrqLimErr1/1 -> [FId_EngDemTrqLimErr1]
  DSM_bEngDemTrqLimErr2/1 -> [FId_EngDemTrqLimErr2]
  DSM_bEngDemTrqLimErr3/1 -> [FId_EngDemTrqLimErr3]
  DSM_bEngDemTrqLimErr4/1 -> [FId_EngDemTrqLimErr4]

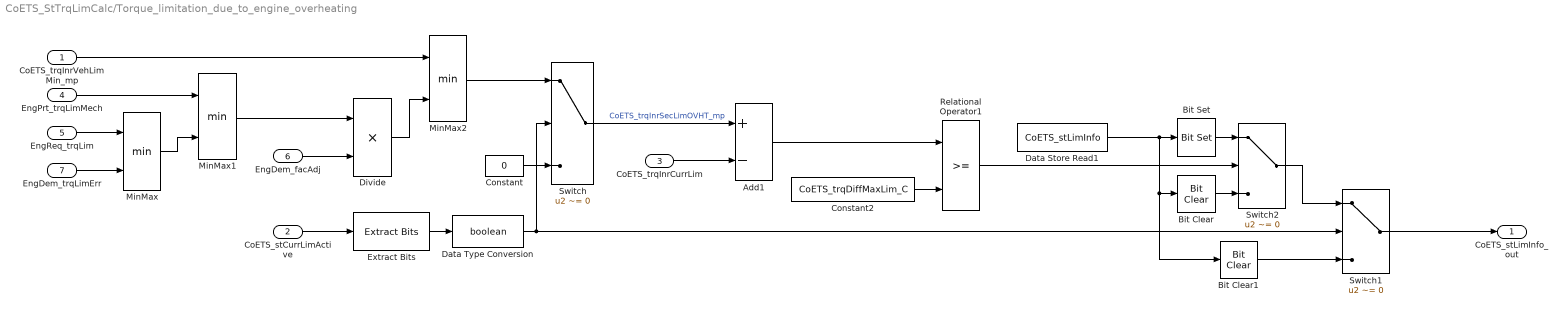
== system CoETS_StTrqLimCalc/Torque_limitation_due_to_engine_overheating ==
  CoETS_trqInrVehLimMin_mp : Inport
  CoETS_stCurrLimActive : Inport  Port=2
  CoETS_trqInrCurrLim : Inport  Port=3
  EngPrt_trqLimMech : Inport  Port=4
  EngReq_trqLim : Inport  Port=5
  EngDem_facAdj : Inport  Port=6
  EngDem_trqLimErr : Inport  Port=7
  Add1 : Sum  Inputs=+-  OutDataTypeStr=Inherit: Inherit via back propagation  SaturateOnIntegerOverflow=on  InputSameDT=on
  Bit Clear : simulink/Logic and Bit Operations/Bit Clear  iBit=0
  Bit Clear1 : simulink/Logic and Bit Operations/Bit Clear  iBit=0
  Bit Set : simulink/Logic and Bit Operations/Bit Set  iBit=0
  Constant : Constant  Value=0  OutDataTypeStr=Inherit: Inherit via back propagation
  Constant2 : Constant  Value=CoETS_trqDiffMaxLim_C
  Data Store Read1 : DataStoreRead  DataStoreName=CoETS_stLimInfo
  Data Type Conversion : DataTypeConversion  OutDataTypeStr=boolean
  Divide : Product  Inputs=**  OutDataTypeStr=Inherit: Inherit via back propagation  SaturateOnIntegerOverflow=on
  Extract Bits : simulink/Logic and Bit Operations/Extract Bits  bitsToExtract=Range of bits  numBits=8  bitIdxRange=5  outScalingMode=Treat bit field as an integer
  MinMax : MinMax  Inputs=2  SaturateOnIntegerOverflow=on  InputSameDT=on
  MinMax1 : MinMax  Inputs=2  SaturateOnIntegerOverflow=on  InputSameDT=on
  MinMax2 : MinMax  Inputs=2  SaturateOnIntegerOverflow=on  InputSameDT=on
  Relational Operator1 : RelationalOperator  OutDataTypeStr=boolean  RndMeth=Nearest  InputSameDT=on
  Switch : Switch  Criteria=u2 ~= 0  SaturateOnIntegerOverflow=on  InputSameDT=on
  Switch1 : Switch  Criteria=u2 ~= 0  SaturateOnIntegerOverflow=on  InputSameDT=on
  Switch2 : Switch  Criteria=u2 ~= 0  SaturateOnIntegerOverflow=on  InputSameDT=on
  "CoETS_stLimInfo_out " : Outport
  wires:
  CoETS_stCurrLimActive/1 -> Extract Bits/1
  EngPrt_trqLimMech/1 -> MinMax1/1
  MinMax/1 -> MinMax1/2
  MinMax1/1 -> Divide/1
  Divide/1 -> MinMax2/2
  MinMax2/1 -> Switch/1
  CoETS_trqInrCurrLim/1 -> Add1/2
  Add1/1 -> Relational Operator1/1
  Constant2/1 -> Relational Operator1/2
  Switch/1 -> Add1/1  "CoETS_trqInrSecLimOVHT_mp"
  Constant/1 -> Switch/3
  Extract Bits/1 -> Data Type Conversion/1
  Relational Operator1/1 -> Switch2/2
  Bit Set/1 -> Switch2/1
  Bit Clear/1 -> Switch2/3
  Switch2/1 -> Switch1/1
  Bit Clear1/1 -> Switch1/3
  Data Store Read1/1 -> Bit Clear1/1, Bit Clear/1, Bit Set/1
  CoETS_trqInrVehLimMin_mp/1 -> MinMax2/1
  EngDem_facAdj/1 -> Divide/2
  EngReq_trqLim/1 -> MinMax/1
  EngDem_trqLimErr/1 -> MinMax/2
  Switch1/1 -> "CoETS_stLimInfo_out "/1
  Data Type Conversion/1 -> Switch1/2, Switch/2

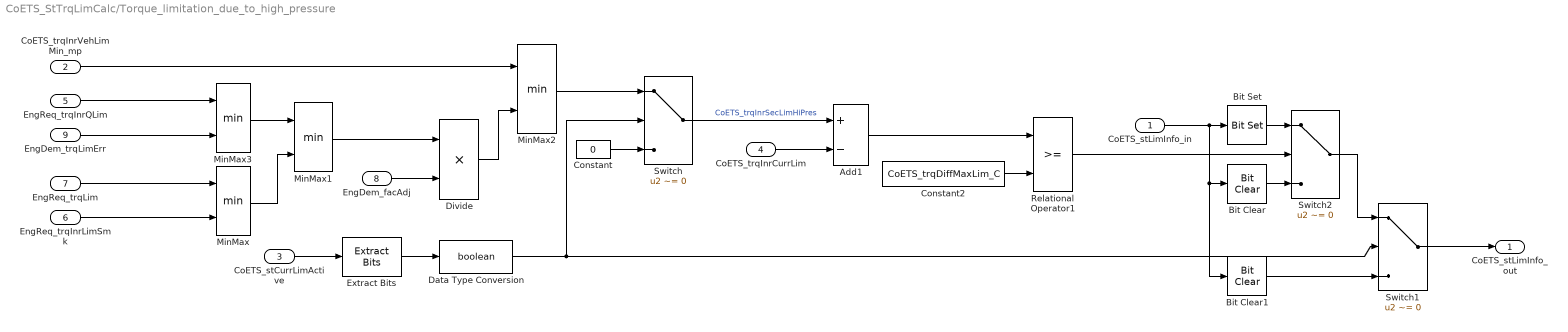
== system CoETS_StTrqLimCalc/Torque_limitation_due_to_high_pressure ==
  CoETS_stLimInfo_in : Inport
  CoETS_trqInrVehLimMin_mp : Inport  Port=2
  CoETS_stCurrLimActive : Inport  Port=3
  CoETS_trqInrCurrLim : Inport  Port=4
  EngReq_trqInrQLim : Inport  Port=5
  EngReq_trqInrLimSmk : Inport  Port=6
  EngReq_trqLim : Inport  Port=7
  EngDem_facAdj : Inport  Port=8
  EngDem_trqLimErr : Inport  Port=9
  Add1 : Sum  Inputs=+-  OutDataTypeStr=Inherit: Inherit via back propagation  InputSameDT=on
  Bit Clear : simulink/Logic and Bit Operations/Bit Clear  iBit=1
  Bit Clear1 : simulink/Logic and Bit Operations/Bit Clear  iBit=1
  Bit Set : simulink/Logic and Bit Operations/Bit Set  iBit=1
  Constant : Constant  Value=0  OutDataTypeStr=Inherit: Inherit via back propagation
  Constant2 : Constant  Value=CoETS_trqDiffMaxLim_C
  Data Type Conversion : DataTypeConversion  OutDataTypeStr=boolean
  Divide : Product  Inputs=**  OutDataTypeStr=Inherit: Inherit via back propagation  SaturateOnIntegerOverflow=on
  Extract Bits : simulink/Logic and Bit Operations/Extract Bits  bitsToExtract=Range of bits  numBits=8  bitIdxRange=9  outScalingMode=Treat bit field as an integer
  MinMax{,1..3} (4 alike) : MinMax  Inputs=2  SaturateOnIntegerOverflow=on  InputSameDT=on
  Relational Operator1 : RelationalOperator  OutDataTypeStr=boolean  RndMeth=Nearest  InputSameDT=on
  Switch : Switch  Criteria=u2 ~= 0  SaturateOnIntegerOverflow=on  InputSameDT=on
  Switch1 : Switch  Criteria=u2 ~= 0  SaturateOnIntegerOverflow=on  InputSameDT=on
  Switch2 : Switch  Criteria=u2 ~= 0  SaturateOnIntegerOverflow=on  InputSameDT=on
  "CoETS_stLimInfo_out " : Outport
  wires:
  Switch1/1 -> "CoETS_stLimInfo_out "/1
  CoETS_stLimInfo_in/1 -> Bit Set/1, Bit Clear/1, Bit Clear1/1
  Bit Clear1/1 -> Switch1/3
  Switch2/1 -> Switch1/1
  Bit Clear/1 -> Switch2/3
  Bit Set/1 -> Switch2/1
  Relational Operator1/1 -> Switch2/2
  Constant/1 -> Switch/3
  Switch/1 -> Add1/1  "CoETS_trqInrSecLimHiPres"
  Constant2/1 -> Relational Operator1/2
  Add1/1 -> Relational Operator1/1
  CoETS_trqInrCurrLim/1 -> Add1/2
  MinMax2/1 -> Switch/1
  Divide/1 -> MinMax2/2
  CoETS_trqInrVehLimMin_mp/1 -> MinMax2/1
  EngDem_facAdj/1 -> Divide/2
  MinMax1/1 -> Divide/1
  MinMax/1 -> MinMax1/2
  EngReq_trqInrQLim/1 -> MinMax3/1
  EngReq_trqInrLimSmk/1 -> MinMax/2
  EngReq_trqLim/1 -> MinMax/1
  CoETS_stCurrLimActive/1 -> Extract Bits/1
  MinMax3/1 -> MinMax1/1
  EngDem_trqLimErr/1 -> MinMax3/2
  Extract Bits/1 -> Data Type Conversion/1
  Data Type Conversion/1 -> Switch/2, Switch1/2

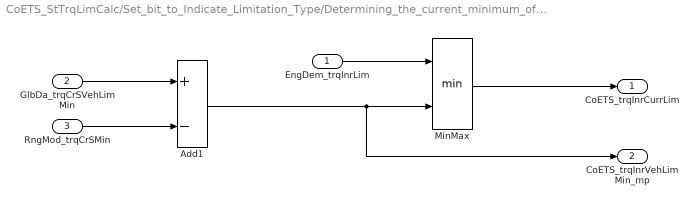
== system CoETS_StTrqLimCalc/Set_bit_to_Indicate_Limitation_Type/Determining_the_current_minimum_of_all_torque_limitations ==
  EngDem_trqInrLim : Inport
  GlbDa_trqCrSVehLimMin : Inport  Port=2
  RngMod_trqCrSMin : Inport  Port=3
  Add1 : Sum  Inputs=+-  OutDataTypeStr=Inherit: Inherit via back propagation  SaturateOnIntegerOverflow=on  InputSameDT=on
  MinMax : MinMax  Inputs=2  SaturateOnIntegerOverflow=on  InputSameDT=on
  CoETS_trqInrCurrLim : Outport
  CoETS_trqInrVehLimMin_mp : Outport  Port=2
  wires:
  MinMax/1 -> CoETS_trqInrCurrLim/1
  Add1/1 -> CoETS_trqInrVehLimMin_mp/1, MinMax/2
  RngMod_trqCrSMin/1 -> Add1/2
  EngDem_trqInrLim/1 -> MinMax/1
  GlbDa_trqCrSVehLimMin/1 -> Add1/1
